simulink model "LK_sim"  (R2025a)
settings: Solver=VariableStepAuto  StartTime=0.0  StopTime=8  RelTol=1e-3
values from neighbouring files (symbols this model uses):
  A = [0 0 0 0 1 -5.61939393939 0 0.163469096877 25 0 0 0 ... (16 elements, 4x4)]    [LK_data.mat]
  B = [0  0; 80.6060606061  0; 0  -1; 63.7627953181  0]    [LK_data.mat]
  nu = 1    [ACC_data.mat]    (also in LK_data.mat)
  nx = 2    [ACC_data.mat]    (also in EstimateUncertaintyBoundsFromData.m = size(X0, 1); LK_data.mat = 4)
  nz = 1    [ACC_data.mat]    (also in EstimateUncertaintyBoundsFromData.m = size(Z0, 1); LK_data.mat)
  T = 0.2    [ACC_data.mat]    (also in LK_data.mat = 0.1)
  x0 = [79.6587016222 17.5244144376]    [ACC_data.mat]
undefined symbols (not defined in the file or in its folder): zk
settings Model: SetupFcn=setupFcn  SimulationMode=accelerator  Creator=12775  LastModifiedBy=12775
settings ModelReferenceCC: EnableRefExpFcnMdlSchedulingChecks=on  EnableParallelModelReferenceBuilds=on  ParallelModelReferenceMATLABWorkerInit=Load Top Model  SupportModelReferenceSimTargetCustomCode=on

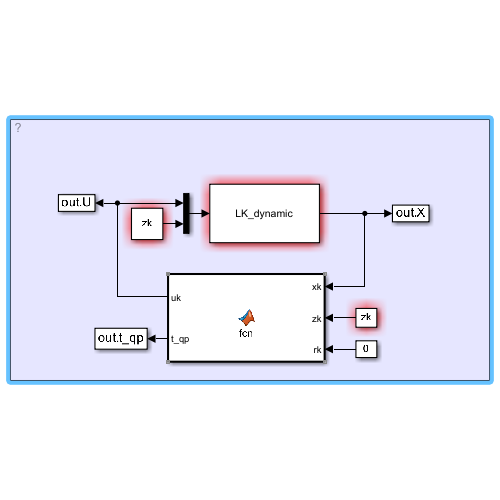
[thumbnail: Simulink's stored preview of the top-level diagram]
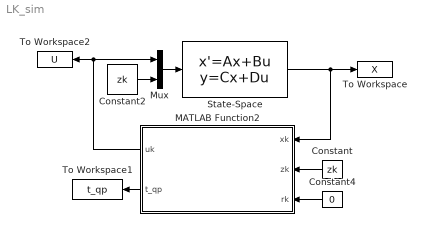
== system LK_sim ==
  Constant : Constant  Value=zk  SampleTime=T
  Constant2 : Constant  Value=zk  SampleTime=T
  Constant4 : Constant  Value=0  SampleTime=T
  MATLAB Function2 : MATLAB Function  TreatAsAtomicUnit=on  SystemSampleTime=T
      settings: MinAlgLoopOccurrences=on
  Mux : Mux  Inputs=2
  State-Space : StateSpace  A=A  B=B  C=eye(nx)  D=zeros(nx,nu+nz)  InitialCondition=x0
      mask DialogControl ParameterGroupVar Prompt: 参数
      mask Display: disp('LK_dynamic');
  To Workspace : ToWorkspace  VariableName=X  SaveFormat=Structure With Time  SampleTime=T
  To Workspace1 : ToWorkspace  VariableName=t_qp  SaveFormat=Structure With Time  SampleTime=T
  To Workspace2 : ToWorkspace  VariableName=U  SaveFormat=Structure With Time  SampleTime=T
  wires:
  Constant/1 -> MATLAB Function2/2(zk)
  Constant2/1 -> Mux/2
  MATLAB Function2/1(uk) -> Mux/1, To Workspace2/1
  State-Space/1 -> To Workspace/1, MATLAB Function2/1(xk)
  Mux/1 -> State-Space/1
  Constant4/1 -> MATLAB Function2/3(rk)
  MATLAB Function2/2(t_qp) -> To Workspace1/1

== matlab function LK_sim/MATLAB Function2 ==
  data: uk output; xk input; zk input; rk input; t_qp output
function [uk, t_qp] = fcn(xk,zk,rk)

coder.extrinsic('evalin');

persistent Controller

if isempty(Controller)
    Controller = evalin('base','Ctrl');
end

uk = 0;                   

tStart = tic;
    uk = Controller(xk,zk,rk);
t_qp = toc(tStart);      

if isnan(uk)
    uk=0;
end

end
